simulink model "Fuzzy_controler"  (R2022b)
settings: Solver=VariableStepAuto  StartTime=0.0  StopTime=299400  RelTol=1e-3
values from neighbouring files (symbols this model uses):
  air_den = 1.225    [wind_turbine_parameters.m]
  l1 = 56    [wind_turbine_parameters.m]
libraries: simulink x1, fuzblock x1
settings Model: Creator=luan  LastModifiedBy=bedat
settings DebuggingCC: AlgebraicLoopMsg=none

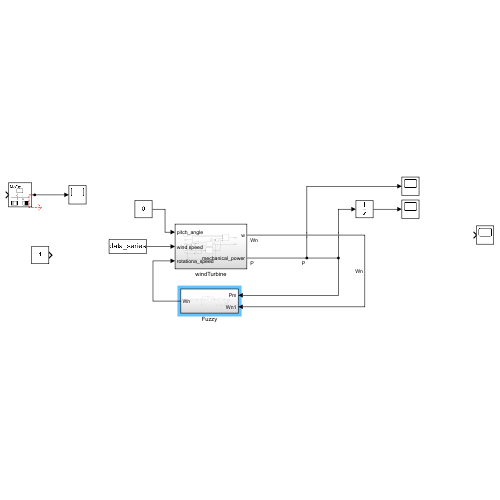
[thumbnail: Simulink's stored preview of the top-level diagram]
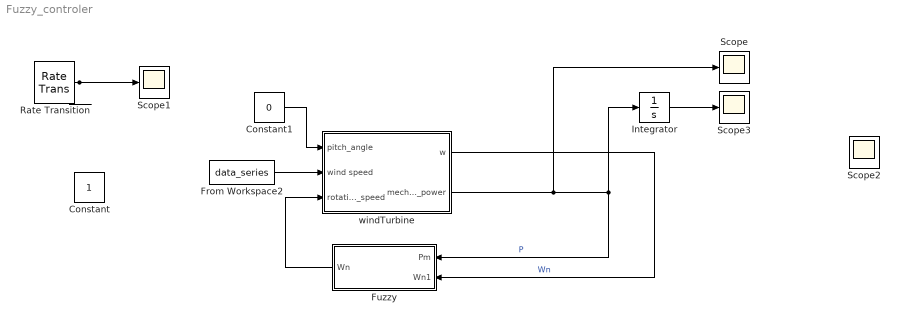
== system Fuzzy_controler ==
  Constant : Constant
  Constant1 : Constant  Value=0
  From Workspace2 : FromWorkspace  VariableName=data_series  SampleTime=600  OutputAfterFinalValue=Holding final value
  Fuzzy : Subsystem
  Integrator : Integrator
  Rate Transition : RateTransition  OutPortSampleTime=600
  Scope{,1..3} (4 alike) : Scope
  windTurbine : Subsystem
  wires:
  From Workspace2/1 -> windTurbine/2(wind speed)
  Constant1/1 -> windTurbine/1(pitch_angle)
  Fuzzy/1(Wn) -> windTurbine/3(rotationa_speed)
  windTurbine/2(mechanical_power) -> Scope/1, Fuzzy/1(Pm), Integrator/1  "P"
  windTurbine/1(w) -> Fuzzy/2(Wn1)  "Wn"
  Integrator/1 -> Scope3/1
  Rate Transition/1 -> Scope1/1

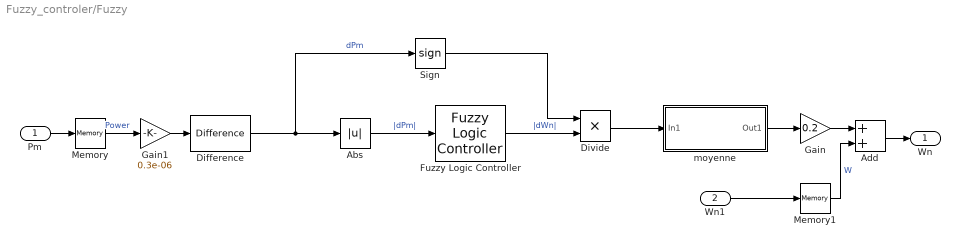
== system Fuzzy_controler/Fuzzy ==
  Pm : Inport
  Wn1 : Inport  Port=2
  Abs : Abs  SaturateOnIntegerOverflow=off
  Add : Sum
  Difference : simulink/Discrete/Difference  ICPrevInput=0.0  OutMin=[]  OutMax=[]  OutDataType=fixdt(1, 16)  OutScaling=2^-10  DoSatur=off
  Divide : Product  Inputs=**
  Fuzzy Logic Controller : fuzblock/Fuzzy Logic  Controller  FIS='version1.fis'  OutputSampleNumber=101  DataType=double  FuzzifiedInputs=off  RuleFiringStrengths=off  RuleOutputs=off  AggregatedOutputs=off  SimulateUsing=Interpreted execution  OutOfRangeInputValueMessage=warning  NoRuleFiredMessage=warning  EmptyOutputFuzzySetMessage=warning
  Gain : Gain  Gain=0.2
  Gain1 : Gain  Gain=0.3e-06
  Memory : Memory
  Memory1 : Memory  InitialCondition=0.2
  Sign : Signum
  moyenne : Subsystem
  Wn : Outport
  wires:
  Abs/1 -> Fuzzy Logic Controller/1  "|dPm|"
  Add/1 -> Wn/1
  Difference/1 -> Sign/1, Abs/1  "dPm"
  Sign/1 -> Divide/1
  Fuzzy Logic Controller/1 -> Divide/2  "|dWn|"
  Divide/1 -> moyenne/1(In1)
  moyenne/1(Out1) -> Gain/1
  Gain/1 -> Add/1
  Gain1/1 -> Difference/1
  Memory1/1 -> Add/2  "W"
  Memory/1 -> Gain1/1  "Power"
  Pm/1 -> Memory/1
  Wn1/1 -> Memory1/1

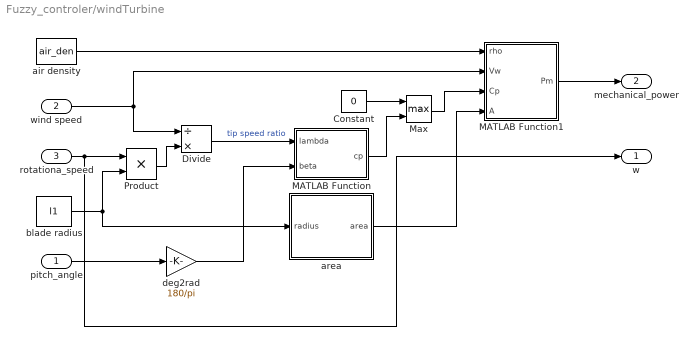
== system Fuzzy_controler/windTurbine ==
  pitch_angle : Inport
  wind speed : Inport  Port=2
  rotationa_speed : Inport  Port=3
  Constant : Constant  Value=0
  Divide : Product  Inputs=/*
  MATLAB Function : MATLAB Function  TreatAsAtomicUnit=on
  MATLAB Function1 : MATLAB Function  TreatAsAtomicUnit=on
  Max : MinMax  Function=max  Inputs=2
  Product : Product
  air density : Constant  Value=air_den
  area : Subsystem
  blade radius : Constant  Value=l1
  deg2rad : Gain  Gain=180/pi
  w : Outport
  mechanical_power : Outport  Port=2
  wires:
  Product/1 -> Divide/2
  wind speed/1 -> Divide/1, MATLAB Function1/2(Vw)
  Divide/1 -> MATLAB Function/1(lambda)  "tip speed ratio"
  pitch_angle/1 -> deg2rad/1
  MATLAB Function1/1(Pm) -> mechanical_power/1
  rotationa_speed/1 -> w/1, Product/1
  air density/1 -> MATLAB Function1/1(rho)
  area/1(area) -> MATLAB Function1/4(A)
  blade radius/1 -> Product/2, area/1(radius)
  deg2rad/1 -> MATLAB Function/2(beta)
  Max/1 -> MATLAB Function1/3(Cp)
  MATLAB Function/1(cp) -> Max/2
  Constant/1 -> Max/1

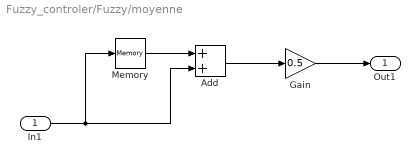
== system Fuzzy_controler/Fuzzy/moyenne ==
  In1 : Inport
  Add : Sum
  Gain : Gain  Gain=0.5
  Memory : Memory
  Out1 : Outport
  wires:
  In1/1 -> Memory/1, Add/2
  Memory/1 -> Add/1
  Add/1 -> Gain/1
  Gain/1 -> Out1/1

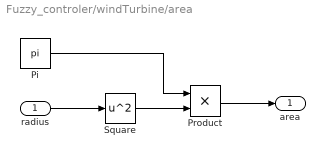
== system Fuzzy_controler/windTurbine/area ==
  radius : Inport
  Pi : Constant  Value=pi  OutDataTypeStr=Inherit: Inherit via back propagation
  Product : Product
  Square : Math  Operator=square
  area : Outport
  wires:
  radius/1 -> Square/1
  Square/1 -> Product/2
  Pi/1 -> Product/1
  Product/1 -> area/1

== matlab function Fuzzy_controler/windTurbine/MATLAB Function ==
  data: lambda input; cp output; beta input
function cp = fcn(lambda, beta)

k = load('coefficients.mat');
lambda_i =  1/(1/(lambda + 0.08*beta) - 0.035/(1+beta*beta*beta));

% Debug
% lambda_i
% k.k1 *(k.k2/lambda_i - k.k3*beta - k.k4*power(beta, k.k5) -k.k6)*exp(-k.k7/lambda_i)

cp = k.k1 *(k.k2/lambda_i - k.k3*beta - k.k4*power(beta, k.k5) -k.k6)*exp(-k.k7/lambda_i);

== matlab function Fuzzy_controler/windTurbine/MATLAB Function1 ==
  data: rho input; Vw input; Pm output; Cp input; A input
function Pm = fcn(rho, Vw, Cp, A)

Pm = 0.5* Cp* rho* A* power(Vw, 3);
